simulink model "maxVelocity"  (R2019a)
settings: Solver=FixedStepAuto  StartTime=0.0  StopTime=inf  FixedStep=1  RelTol=1e-3
values from neighbouring files (symbols this model uses):
  init =     [course_data_0_1m.mat]
libraries: simulink x2
settings Model: Creator=Frieder Uerlings  LastModifiedBy=Frieder Uerlings
settings DataIOCC: SaveFinalState=on

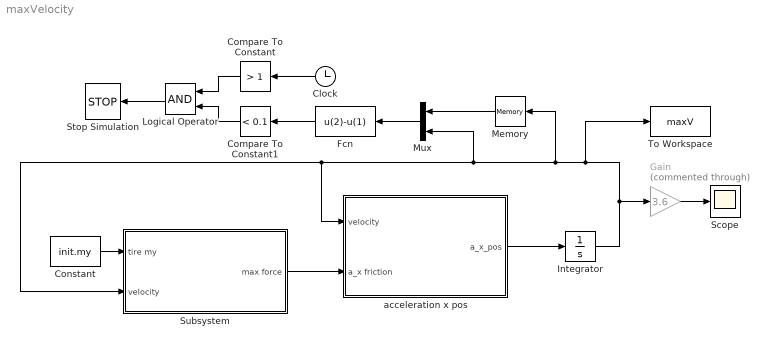
== system maxVelocity ==
  Clock : Clock
  Compare To Constant : simulink/Logic and Bit Operations/Compare To Constant  relop=>  const=1  OutDataTypeStr=boolean
  Compare To Constant1 : simulink/Logic and Bit Operations/Compare To Constant  relop=<  const=0.1  OutDataTypeStr=boolean
  Constant : Constant  Value=init.my
  Fcn : Fcn  Expr=u(2)-u(1)
  Gain : Gain  Commented=through  Gain=3.6
  Integrator : Integrator
  Logical Operator : Logic  AllPortsSameDT=off  OutDataTypeStr=boolean
  Memory : Memory
  Mux : Mux  Inputs=2
  Scope : Scope
  Stop Simulation : Stop
  Subsystem : Subsystem
  To Workspace : ToWorkspace  VariableName=maxV  SampleTime=-1
  acceleration x pos : Subsystem
  wires:
  acceleration x pos/1("a_x_pos ") -> Integrator/1
  Subsystem/1(max force) -> acceleration x pos/2(a_x friction)
  Constant/1 -> Subsystem/1(tire my)
  Integrator/1 -> To Workspace/1, Memory/1, Mux/2, Subsystem/2(velocity), acceleration x pos/1(velocity), Gain/1
  Memory/1 -> Mux/1
  Mux/1 -> Fcn/1
  Clock/1 -> Compare To Constant/1
  Fcn/1 -> Compare To Constant1/1
  Compare To Constant1/1 -> Logical Operator/2
  Compare To Constant/1 -> Logical Operator/1
  Logical Operator/1 -> Stop Simulation/1
  Gain/1 -> Scope/1

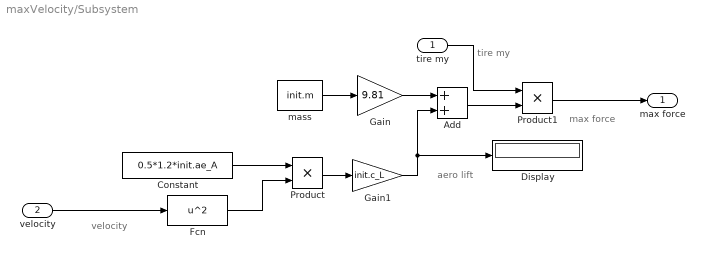
== system maxVelocity/Subsystem ==
  note: max force
  note: aero lift
  note: tire my
  note: velocity
  tire my : Inport
  velocity : Inport  Port=2
  Add : Sum
  Constant : Constant  Value=0.5*1.2*init.ae_A
  Display : Display
  Fcn : Fcn  Expr=u^2
  Gain : Gain  Gain=9.81
  Gain1 : Gain  Gain=init.c_L
  Product : Product
  Product1 : Product
  "mass " : Constant  Value=init.m
  max force : Outport
  wires:
  Constant/1 -> Product/1
  Add/1 -> Product1/2
  "mass "/1 -> Gain/1
  Fcn/1 -> Product/2
  Product1/1 -> max force/1
  Gain/1 -> Add/1
  Product/1 -> Gain1/1
  tire my/1 -> Product1/1
  velocity/1 -> Fcn/1
  Gain1/1 -> Add/2, Display/1

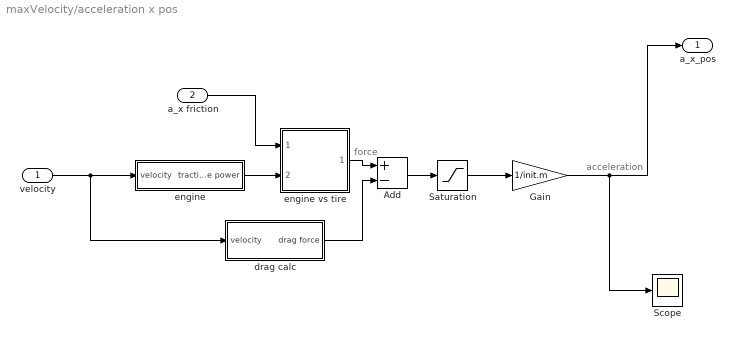
== system maxVelocity/acceleration x pos ==
  note: force
  note: acceleration
  velocity : Inport
  a_x friction : Inport  Port=2
  Add : Sum  Inputs=+-
  Gain : Gain  Gain=1/init.m
  Saturation : Saturate  UpperLimit=inf  LowerLimit=0
  Scope : Scope
  drag calc : Subsystem
  engine : Subsystem
  engine vs tire : Subsystem
  "a_x_pos " : Outport
  wires:
  engine vs tire/1(acc force) -> Add/1
  Gain/1 -> "a_x_pos "/1, Scope/1
  Add/1 -> Saturation/1
  drag calc/1("drag force ") -> Add/2
  engine/1(tractive power) -> engine vs tire/2(tractive power)
  a_x friction/1 -> engine vs tire/1("a_x friction ")
  velocity/1 -> drag calc/1(velocity), engine/1(velocity)
  Saturation/1 -> Gain/1

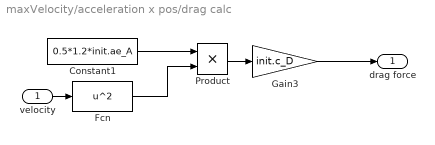
== system maxVelocity/acceleration x pos/drag calc ==
  velocity : Inport
  Constant1 : Constant  Value=0.5*1.2*init.ae_A
  Fcn : Fcn  Expr=u^2
  Gain3 : Gain  Gain=init.c_D
  Product : Product
  "drag force " : Outport
  wires:
  Constant1/1 -> Product/1
  velocity/1 -> Fcn/1
  Fcn/1 -> Product/2
  Product/1 -> Gain3/1
  Gain3/1 -> "drag force "/1

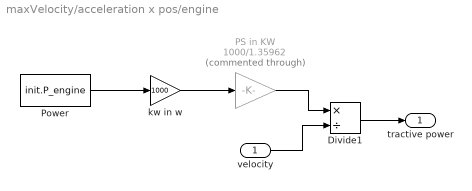
== system maxVelocity/acceleration x pos/engine ==
  velocity : Inport
  Divide1 : Product  Inputs=*/
  "PS in KW " : Gain  Commented=through  Gain=1000/1.35962
  "Power " : Constant  Value=init.P_engine
  "kw in w " : Gain  Gain=1000
  tractive power : Outport
  wires:
  "Power "/1 -> "kw in w "/1
  "PS in KW "/1 -> Divide1/1
  Divide1/1 -> tractive power/1
  velocity/1 -> Divide1/2
  "kw in w "/1 -> "PS in KW "/1

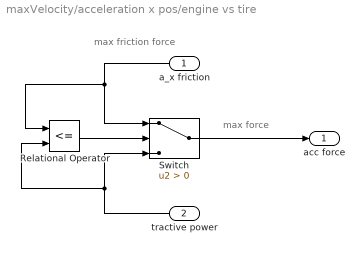
== system maxVelocity/acceleration x pos/engine vs tire ==
  note: max force
  note: max friction force
  "a_x friction " : Inport
  tractive power : Inport  Port=2
  Relational Operator : RelationalOperator  Operator=<=  OutDataTypeStr=boolean  RndMeth=Simplest
  Switch : Switch  Criteria=u2 > Threshold
  acc force : Outport
  wires:
  tractive power/1 -> Relational Operator/2, Switch/3
  "a_x friction "/1 -> Relational Operator/1, Switch/1
  Switch/1 -> acc force/1
  Relational Operator/1 -> Switch/2
